simulink model "openMHA_test_FIFO"  (R2020a)
settings: Solver=VariableStepAuto  StartTime=0.0  StopTime=18  RelTol=1e-3
libraries: dspsrcs4 x3, hdlsllib x1
settings Model: Creator=t96f346  LastModifiedBy=t96f346

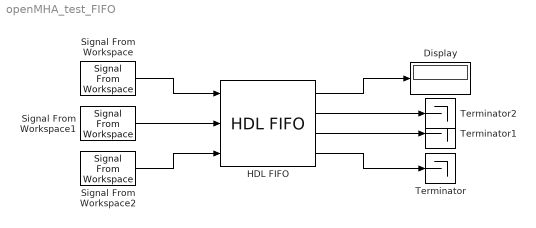
== system openMHA_test_FIFO ==
  Display : Display
  HDL FIFO : hdlsllib/HDL RAMs/HDL FIFO  fifo_size=18  mode=Classic  ratio=1  push_msg=Warning  pop_msg=Warning  show_empty=on  show_full=on  show_num=on  LabelModeActiveChoice_Mode=Classic
      settings: SourceProductBaseCode=SL
  Signal From Workspace : dspsrcs4/Signal From Workspace  X=in  Ts=1  nsamps=1  OutputAfterFinalValue=Setting to zero  ignoreOrWarnInputAndFrameLengths=off  OutputFrames=off
  Signal From Workspace1 : dspsrcs4/Signal From Workspace  X=push  Ts=1  nsamps=1  OutputAfterFinalValue=Setting to zero  ignoreOrWarnInputAndFrameLengths=off  OutputFrames=off
  Signal From Workspace2 : dspsrcs4/Signal From Workspace  X=pop  Ts=1  nsamps=1  OutputAfterFinalValue=Setting to zero  ignoreOrWarnInputAndFrameLengths=off  OutputFrames=off
  Terminator : Terminator
  Terminator1 : Terminator
  Terminator2 : Terminator
  wires:
  Signal From Workspace/1 -> HDL FIFO/1
  Signal From Workspace1/1 -> HDL FIFO/2
  Signal From Workspace2/1 -> HDL FIFO/3
  HDL FIFO/1 -> Display/1
  HDL FIFO/4 -> Terminator/1
  HDL FIFO/3 -> Terminator1/1
  HDL FIFO/2 -> Terminator2/1
